simulink model "main"  (R2017a)
settings: Solver=VariableStepAuto  StartTime=0.0  StopTime=10.0  RelTol=1e-3
values from neighbouring files (symbols this model uses):
  curve_fit = [ 0 0;               0 0;               0 0;               0 0;               0 0;               0 0;               0 0;               0 0;               0 0]    [main.m]
  freq = [ 0; 0; 0; 0; 0; 0; 0; 0; 0]    [main.m]
  pulse_width = [ 0; 0; 0; 0; 0; 0; 0; 0; 0]    [main.m]
settings Model: Creator=Nathaniel  LastModifiedBy=Nathaniel

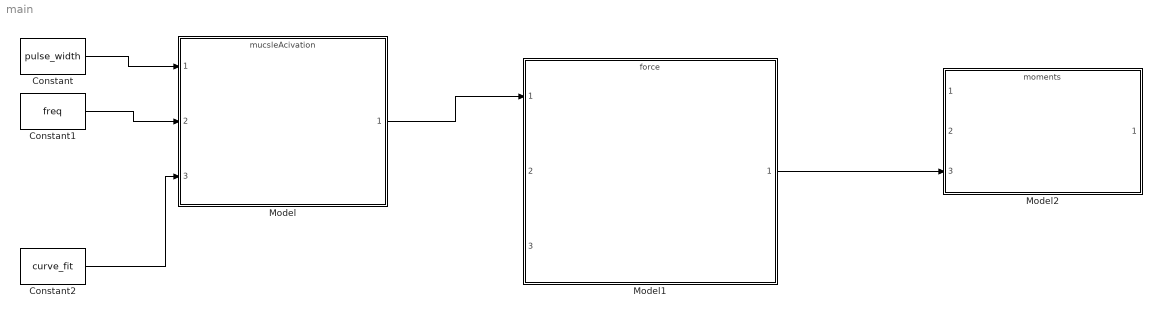
== system main ==
  Constant : Constant  Value=pulse_width
  Constant1 : Constant  Value=freq
  Constant2 : Constant  Value=curve_fit
  Model : ModelReference  ModelNameDialog=mucsleAcivation.slx  SimulationMode=Normal  ModelReferenceVersion=1.12
  Model1 : ModelReference  ModelNameDialog=force.slx  SimulationMode=Normal  ModelReferenceVersion=1.9
  Model2 : ModelReference  ModelNameDialog=moments.slx  SimulationMode=Normal  ModelReferenceVersion=1.4
  wires:
  Constant/1 -> Model/1
  Constant1/1 -> Model/2
  Constant2/1 -> Model/3
  Model/1 -> Model1/1
  Model1/1 -> Model2/3
